simulink model "Automated_Inputs"  (R2022a)
settings: Solver=VariableStepAuto  StartTime=0.0  StopTime=10.0  RelTol=1e-3
undefined symbols (not defined in the file): Freq_Sine, period, pulse_width
settings Model: Creator=chadw  LastModifiedBy=chadw

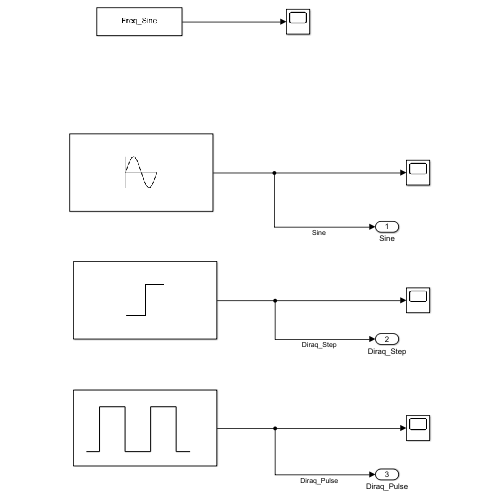
[thumbnail: Simulink's stored preview of the top-level diagram]
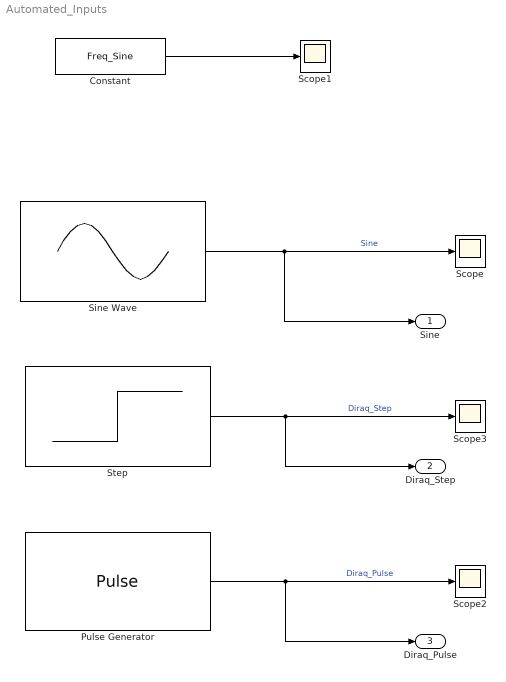
== system Automated_Inputs ==
  Constant : Constant  Value=Freq_Sine
  Pulse Generator : DiscretePulseGenerator  PulseType=Time based  Period=period  PulseWidth=pulse_width
  Scope{,1..3} (4 alike) : Scope
  Sine Wave : Sin  Frequency=Freq_Sine  SampleTime=0
  Step : Step  SampleTime=0
  Sine : Outport
  Diraq_Step : Outport  Port=2
  Diraq_Pulse : Outport  Port=3
  wires:
  Sine Wave/1 -> Sine/1, Scope/1  "Sine"
  Constant/1 -> Scope1/1
  Pulse Generator/1 -> Diraq_Pulse/1, Scope2/1  "Diraq_Pulse"
  Step/1 -> Diraq_Step/1, Scope3/1  "Diraq_Step"
